simulink model "pitch_attitude_hold"  (Simulink 7.7)
settings: Solver=ode3  StartTime=0.0  StopTime=10.0  RelTol=1e-3
undefined symbols (not defined in the file): a_theta_1, a_theta_2, a_theta_3, k_d_theta, k_p_theta
settings Model: Creator=prattmic  LastModifiedBy=prattmic
settings OptimizationCC: InlineParams=on
settings HardwareCC: ProdLargestAtomicInteger=Long  ProdLargestAtomicFloat=Double  ProdEndianess=LittleEndian  ProdHWDeviceType=ARM Compatible->ARM Cortex

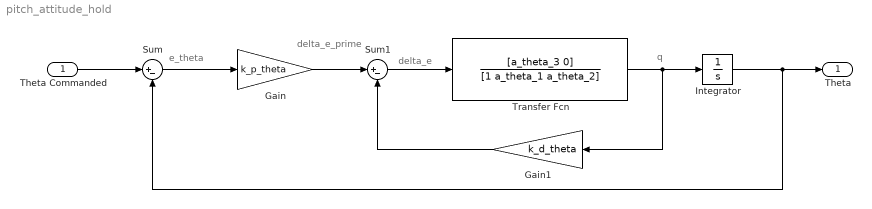
== system pitch_attitude_hold ==
  note: e_theta
  note: delta_e_prime
  note: delta_e
  note: q
  Theta Commanded : Inport
  Gain : Gain  Gain=k_p_theta
  Gain1 : Gain  Gain=k_d_theta
  Integrator : Integrator
  Sum : Sum  Inputs=|+-
  Sum1 : Sum  Inputs=|+-
  Transfer Fcn : TransferFcn  Numerator=[a_theta_3 0]  Denominator=[1 a_theta_1 a_theta_2]
  Theta : Outport
  wires:
  Theta Commanded/1 -> Sum/1
  Sum/1 -> Gain/1
  Gain/1 -> Sum1/1
  Sum1/1 -> Transfer Fcn/1
  Integrator/1 -> Theta/1, Sum/2
  Gain1/1 -> Sum1/2
  Transfer Fcn/1 -> Integrator/1, Gain1/1
